simulink library "gavrt_library"  (Simulink 7.1)
undefined symbols (not defined in the file or in its folder): Convert, Counter, Mux, xbsIndex_r3
libraries: xbsIndex_r4 x210, xps_library x15, casper_library x12, gavrt_library x8, xbsReplacements_r4 x7
(part 2 of 3)

== system gavrt_library/commutator ==
  reset : Inport  OutDataType=sfix(16)  OutScaling=2^0
  enable : Inport  Port=2  OutDataType=sfix(16)  OutScaling=2^0
  din : Inport  Port=3  OutDataType=sfix(16)  OutScaling=2^0
  Mux : S-Function  AncestorBlock=xbsIndex_r3/Mux  FunctionName=xlmux  Parameters=sfcn_mwsv__  EnableBusSupport=off  mask(Xilinx Multiplexer Block){inputs=8, precision=Full, arith_type=Signed  (2's comp), n_bits=8, bin_pt=2, quantization=Truncate, overflow=Wrap, latency=2, explicit_period=off, period=1, en=off, dbl_ovrd=off, show_param=off, mux_type=off, use_rpm=off, gen_core=off, xl_area=[0, 0, 0, 0, 0, 0, 0], xl_use_area=off}
      mask prompts: inputs "Number of Inputs"; arith_type "Arithmetic Type"; n_bits "Number of Bits"; bin_pt "Binary Point"; explicit_period "Use Explicit Sample Period"; period "Sample Period  (use -1 to inherit first known input period)"; en "Provide Enable Port"; dbl_ovrd "Override with Doubles"; show_param "---------------------- Show Implementation Parameters -----------------------------------------------------------------------------------"; mux_type "Use Tristate Buffers"; use_rpm "Use Placement Information for Core"; gen_core "Generate Core"; xl_area "FPGA Area [Slices, FFs, BRAMs, LUTs, IOBs, Emb. Mults, TBUFs]"; xl_use_area "Use Area Above For Estimation"
      mask help:
      | Bus Multiplexer.  Binary points are aligned automatically.
      |
      | Hardware notes: A multiplexer using tristate buffers requires fewer lookup tables but is slower.
      mask init:
      | [designRoot, family, part, speed, package, simulinkPeriod, sysclkPeriod, dbl_ovrd, trimVbit] = xlSysgenSettings(gcb,1,1);
      | num_inputs = inputs+1;
      | [bg,fg] = xlcmap('XBlock',dbl_ovrd);
      | zstr='';
      | zpstr='';
      | if latency > 0
      |   zstr = 'z';
      |   zpstr = sprintf('-%d', latency);
      | end
      | 
      | dprt = [2:inputs+2 2+zeros(1,32-inputs)];
      | dstr0 = 'd0';
      | dstr1 = 'd1';
      | dstr2='';dstr3='';dstr4='';dstr5='';dstr6='';dstr7='';dstr8='';dstr9='';dstr10='';
      | dstr11='';dstr12='';dstr12='';dstr13='';dstr14='';dstr15='';dstr16='';dstr17='';dstr18='';dstr19='';dstr20='';dstr21='';dstr22='';dstr23='';dstr24='';dstr25='';dstr26='';dstr27='';dstr28='';dstr29='';dstr30='';dstr31='';
      | 
      | if (inputs>=2) dstr2 = 'd2'; end
      | if (inputs>=3) dstr3 = 'd3'; end
      | if (inputs>=4) dstr4 = 'd4'; end
      | if (inputs>=5) dstr5 = 'd5'; end
      | if (inputs>=6) dstr6 = 'd6'; end
      | if (inputs>=7) dstr7 = 'd7'; end
      | if (inputs>=8) dstr8 = 'd8'; end
      | if (inputs>=9) dstr9 = 'd9'; end
      | if (inputs>=10) dstr10 = 'd10'; end
      | if (inputs>=11) dstr11 = 'd11'; end
      | if (inputs>=12) dstr12 = 'd12'; end
      | if (inputs>=13) dstr13 = 'd13'; end
      | if (inputs>=14) dstr14 = 'd14'; end
      | if (inputs>=15) dstr15 = 'd15'; end
      | if (inputs>=16) dstr16 = 'd16'; end
      | if (inputs>=17) dstr17 = 'd17'; end
      | if (inputs>=18) dstr18 = 'd18'; end
      | if (inputs>=19) dstr19 = 'd19'; end
      | if (inputs>=20) dstr20 = 'd20'; end
      | if (inputs>=21) dstr21 = 'd21'; end
      | if (inputs>=22) dstr22 = 'd22'; end
      | if (inputs>=23) dstr23 = 'd23'; end
      | if (inputs>=24) dstr24 = 'd24'; end
      | if (inputs>=25) dstr25 = 'd25'; end
      | if (inputs>=26) dstr26 = 'd26'; end
      | if (inputs>=27) dstr27 = 'd27'; end
      | if (inputs>=28) dstr28 = 'd28'; end
      | if (inputs>=29) dstr29 = 'd29'; end
      | if (inputs>=30) dstr30 = 'd30'; end
      | if (inputs>=31) dstr31 = 'd31'; end
      | 
      | iPos = get_param(gcb,'Position');
      | iWidth=iPos(3)-iPos(1); iHeight=iPos(4)-iPos(2);
      | iCx=iWidth/2;
      | iCy=iHeight/2;
      | [logoX, logoY] = xlogo(iPos);
      | 
      | rst = 0;
      | [enPortNum, enPortStr, rstPortNum, rstPortStr, portDir] = xlport_en_rst(en, rst, num_inputs+2);
      | % one time added for param list
      | hasEN = en;
      | hasRST = rst;
      | dblOvrd = dbl_ovrd;
      | numInputs = num_inputs;
      | muxType = mux_type;
      | useCore = 1;
      | precision0 = precision;
      | z0 = [n_bits  bin_pt arith_type quantization overflow];
      | explicitClk = explicit_period;
      | gen_core = 1;
      | 
      | % just pass everything to s-function
      | sfcn_mwsv__ = get_param(gcb, 'MaskWSVariables');
      mask Help: eval('xlWeb(xlhtmldoclink(''Mux''))');
      mask StyleString: popup(2|3|4|5|6|7|8|9|10|11|12|13|14|15|16|17|18|19|20|21|22|23|24|25|26|27|28|29|30|31|32),popup(Full|User Defined),popup(Unsigned|Signed  (2's comp)),edit,edit,popup(Truncate|Round  (unbiased: +/- Inf)),popup(Wrap|Saturate|Flag as Error),edit,checkbox,edit,checkbox,checkbox,checkbox,checkbox,checkbox,checkbox,edit,checkbox
      mask CallbackString: |xlMagicCallback|||||||xlMagicCallback||||xlShowIPCallback|||||
      mask Display:
      | patch([0 iWidth iWidth 0],[0 1/7*iHeight 6/7*iHeight iHeight] , bg);
      | patch(logoX,logoY, fg);
      | plot([0 iWidth iWidth 0 0],[0 1/7*iHeight 6/7*iHeight iHeight 0] );
      | text(iCx-5,iCy-5,zstr);
      | text(iCx,iCy,zpstr);
      | port_label('input',1,'sel');
      | port_label('input',dprt(1),dstr0);
      | port_label('input',dprt(2),dstr1);
      | port_label('input',dprt(2),dstr1);
      | port_label('input',dprt(3),dstr2);
      | port_label('input',dprt(4),dstr3);
      | port_label('input',dprt(5),dstr4);
      | port_label('input',dprt(6),dstr5);
      | port_label('input',dprt(7),dstr6);
      | port_label('input',dprt(8),dstr7);
      | port_label('input',dprt(9),dstr8);
      | port_label('input',dprt(10),dstr9);
      | port_label('input',dprt(11),dstr10);
      | port_label('input',dprt(12),dstr11);
      | port_label('input',dprt(13),dstr12);
      | port_label('input',dprt(14),dstr13);
      | port_label('input',dprt(15),dstr14);
      | port_label('input',dprt(16),dstr15);
      | port_label('input',dprt(17),dstr16);
      | port_label('input',dprt(18),dstr17);
      | port_label('input',dprt(19),dstr18);
      | port_label('input',dprt(20),dstr19);
      | port_label('input',dprt(21),dstr20);
      | port_label('input',dprt(22),dstr21);
      | port_label('input',dprt(23),dstr22);
      | port_label('input',dprt(24),dstr23);
      | port_label('input',dprt(25),dstr24);
      | port_label('input',dprt(26),dstr25);
      | port_label('input',dprt(27),dstr26);
      | port_label('input',dprt(28),dstr27);
      | port_label('input',dprt(29),dstr28);
      | port_label('input',dprt(30),dstr29);
      | port_label('input',dprt(31),dstr30);
      | port_label('input',dprt(32),dstr31);
      | port_label(portDir,enPortNum,enPortStr);
  index_cnt : S-Function  AncestorBlock=xbsIndex_r3/Counter  FunctionName=xlcounter  Parameters=sfcn_mwsv__  EnableBusSupport=off  mask(Xilinx Counter Block){cnt_type=Free Running, n_bits=3, bin_pt=0, arith_type=Unsigned, start_count=0, cnt_to=Inf, cnt_by_val=1, operation=Up, explicit_period=off, period=1, load_pin=off, rst=on, en=on, dbl_ovrd=off, show_param=off, use_rpm=on, gen_core=off, xl_area=[0, 0, 0, 0, 0, 0, 0], xl_use_area=off}
      mask prompts: cnt_type "Counter Type"; n_bits "Number of Bits"; bin_pt "Binary Point Position"; arith_type "Arithmetic Type"; start_count "Initial Value"; cnt_to "Count To Value"; cnt_by_val "Step"; operation "Count Direction"; explicit_period "Use Explicit Sample Period"; period "Sample Period"; load_pin "Provide Load Port"; rst "Provide Reset Port"; en "Provide Enable Port"; dbl_ovrd "Override with Doubles"; show_param "---------------------- Show Implementation Parameters -----------------------------------------------------------------------------------"; use_rpm "Use Placement Information for Core"; gen_core "Generate Core"; xl_area "FPGA Area [Slices, FFs, BRAMs, LUTs, IOBs, Emb. Mults, TBUFs]"; xl_use_area "Use Area Above For Estimation"
      mask help:
      | Configurable up, down and up/down counter.
      |
      | Hardware notes: Free running counters are the least expensive in hardware.  A count limited counter is implemented by combining a counter with a comparator.
      mask init:
      | if ((rst==1) | (en==1) | (operation == 3) | ( (cnt_type == 2)&(load_pin == 1)))
      |   explicitClk = explicit_period;
      | else
      |   explicitClk =1;
      | end
      | numinputs = 0;
      | upDir = 'output';
      | upPNum = 1;
      | upStr = '';
      | loadDir = 'output';
      | loadPNum = 1;
      | loadStr = '';
      | dinDir = 'output';
      | dinPNum = 1;
      | dinStr = '';
      | if (operation == 3)
      |    numinputs = numinputs + 1;
      |    upDir = 'input';
      |   upPNum = numinputs;
      |    upStr = 'up';
      | end
      | 
      | if (cnt_type == 2)
      |   if (load_pin)
      |     loadDir = 'input';
      |     loadStr = 'load';
      |     numinputs = numinputs + 1;
      |     loadPNum = numinputs;
      |     dinDir = 'input';
      |     dinStr = 'din';
      |     numinputs = numinputs + 1;
      |     dinPNum = numinputs;
      |  end
      | end
      | numinputs = numinputs + 1;
      | [designRoot, family, part, speed, package, simulinkPeriod, sysclkPeriod, dbl_ovrd, trimVbit] = xlSysgenSettings(gcb,1,1);
      | [enPortNum, enPortStr, rstPortNum, rstPortStr, portDir] = xlport_en_rst(en, rst, numinputs);
      | [bg,fg]=xlcmap('XBlock',dbl_ovrd);
      | iPos = get_param(gcb,'Position');
      | iWidth=iPos(3)-iPos(1); iHeight=iPos(4)-iPos(2);
      | iCx=iWidth/2;
      | iCy=iHeight/2;
      | [logoX, logoY] = xlogo(iPos);
      | 
      | 
      | % one time added for param list
      | dblOvrd = dbl_ovrd;
      | precision0 = 2;
      | z0 = [n_bits bin_pt arith_type  1 1];
      | hasEN = en;
      | hasRST = rst;
      | hasLoad = load_pin;
      | latency = 1;
      | useCore = 1;
      | gen_core = 1;
      | 
      | % just pass everything to s-function
      | sfcn_mwsv__ = get_param(gcb, 'MaskWSVariables');
      mask Help: eval('xlWeb(xlhtmldoclink(''Counter''))');
      mask StyleString: popup(Count Limited|Free Running),edit,edit,popup(Unsigned|Signed  (2's comp)),edit,edit,edit,popup(Up|Down|Up/Down),checkbox,edit,checkbox,checkbox,checkbox,checkbox,checkbox,checkbox,checkbox,edit,checkbox
      mask CallbackString: xlcounterCallback|||||||xlcounterCallback|xlcounterCallback||xlcounterCallback|xlcounterCallback|xlcounterCallback||xlShowIPCallback||||
      mask Display:
      | patch([0 iWidth iWidth 0],[0 0 iHeight iHeight] , bg);
      | patch(logoX,logoY , fg);
      | port_label('output',1,'out');
      | port_label(upDir,upPNum,upStr);
      | port_label(dinDir,dinPNum,dinStr);
      | port_label(loadDir,loadPNum,loadStr);
      | port_label(portDir,rstPortNum,rstPortStr);
      | port_label(portDir,enPortNum,enPortStr);
      | plot([0 0 iWidth iWidth 0], [0 iHeight iHeight 0 0]);
  uncram : gavrt_library/uncram  SystemSampleTime=-1  num_slice=8  slice_width=32  bin_pt=0  arith_type=0
      settings: AttributesFormatString=UFix_32_0
  index : Outport  Orientation=up  OutDataType=sfix(16)  OutScaling=2^0
  dout : Outport  Port=2  OutDataType=sfix(16)  OutScaling=2^0
  wires:
  reset/1 -> index_cnt/1
  enable/1 -> index_cnt/2
  din/1 -> uncram/1
  index_cnt/1 -> index/1, Mux/1
  Mux/1 -> dout/1
  uncram/1 -> Mux/2
  uncram/2 -> Mux/3
  uncram/3 -> Mux/4
  uncram/4 -> Mux/5
  uncram/5 -> Mux/6
  uncram/6 -> Mux/7
  uncram/7 -> Mux/8
  uncram/8 -> Mux/9

== system gavrt_library/cram ==
  In1 : Inport  OutDataType=sfix(16)  OutScaling=2^0
  In2 : Inport  Port=2  OutDataType=sfix(16)  OutScaling=2^0
  In3 : Inport  Port=3  OutDataType=sfix(16)  OutScaling=2^0
  In4 : Inport  Port=4
  Concat : xbsIndex_r4/Concat  num_inputs=4  dbl_ovrd=off  block_type=concat
      settings: block_version=10.1.2
  Reinterp{1..4} (4 alike) : xbsIndex_r4/Reinterpret  force_arith_type=on  arith_type=Unsigned  force_bin_pt=on  bin_pt=0  block_type=reinterpret
      settings: infoedit="Changes signal type without altering the binary representation.   You can changed the signal between signed and unsigned, and relocate the binary point.<P><P>Hardware notes: In hardware this block costs nothing.<P><P>Example:  Suppose the input is 6 bits wide, signed, with 2 fractional bits, and the output is forced to unsigned with 0 fractional bits.  Then an input of -2.0 (1110.00 in binary 2's complement) becomes an output of 56 (111000 in binary)."  block_version=10.1.2
  Out : Outport
  wires:
  Reinterp4/1 -> Concat/4
  In4/1 -> Reinterp4/1
  Reinterp3/1 -> Concat/3
  In3/1 -> Reinterp3/1
  Reinterp2/1 -> Concat/2
  In2/1 -> Reinterp2/1
  Reinterp1/1 -> Concat/1
  In1/1 -> Reinterp1/1
  Concat/1 -> Out/1

== system gavrt_library/fpga_cplx_to_sim_cplx ==
  in : Inport  OutDataType=sfix(16)  OutScaling=2^0
  Gateway Out10 : xbsIndex_r4/Gateway Out  hdl_port=on  timing_constraint=None  locs_specified=off  LOCs={}  block_type=gatewayout
      settings: infoedit="Gateway out block.  Converts Xilinx fixed point inputs into ouputs of type Simulink integer, double, or fixed point.<P><P>Hardware notes:  In hardware these blocks become top level output ports or are discarded, depending on how they are configured."  xl_area=[0, 0, 0, 0, 0, 0, 0]  block_version=10.1.2
  Gateway Out6 : xbsIndex_r4/Gateway Out  hdl_port=on  timing_constraint=None  locs_specified=off  LOCs={}  block_type=gatewayout
      settings: infoedit="Gateway out block.  Converts Xilinx fixed point inputs into ouputs of type Simulink integer, double, or fixed point.<P><P>Hardware notes:  In hardware these blocks become top level output ports or are discarded, depending on how they are configured."  xl_area=[0, 0, 0, 0, 0, 0, 0]  block_version=10.1.2
  Real-Imag to Complex : RealImagToComplex
  c_to_ri : casper_library/Misc/c_to_ri  SystemSampleTime=-1  n_bits=width  bin_pt=width-1
      settings: AttributesFormatString=18_17 r/i
  cplx : Outport  OutDataType=sfix(16)  OutScaling=2^0
  re : Outport  Port=2  OutDataType=sfix(16)  OutScaling=2^0
  im : Outport  Port=3  OutDataType=sfix(16)  OutScaling=2^0
  wires:
  c_to_ri/1 -> Gateway Out6/1
  c_to_ri/2 -> Gateway Out10/1
  Gateway Out6/1 -> Real-Imag to Complex/1, re/1
  Gateway Out10/1 -> Real-Imag to Complex/2, im/1
  Real-Imag to Complex/1 -> cplx/1
  in/1 -> c_to_ri/1

== system gavrt_library/nCasts ==
  In1 : Inport  OutDataType=sfix(16)  OutScaling=2^0
  In2 : Inport  Port=2  OutDataType=sfix(16)  OutScaling=2^0
  Cast1 : xbsIndex_r4/Convert  arith_type=Unsigned  n_bits=8  bin_pt=3  quantization=Truncate  overflow=Wrap  latency=0  dbl_ovrd=off  pipeline=off  block_type=convert
      settings: xl_area=[0, 0, 0, 0, 0, 0, 0]  block_version=10.1.2
  Cast2 : xbsIndex_r4/Convert  arith_type=Unsigned  n_bits=8  bin_pt=3  quantization=Truncate  overflow=Wrap  latency=0  dbl_ovrd=off  pipeline=off  block_type=convert
      settings: xl_area=[0, 0, 0, 0, 0, 0, 0]  block_version=10.1.2
  Out1 : Outport  OutDataType=sfix(16)  OutScaling=2^0
  Out2 : Outport  Port=2  OutDataType=sfix(16)  OutScaling=2^0
  wires:
  Cast2/1 -> Out2/1
  In2/1 -> Cast2/1
  Cast1/1 -> Out1/1
  In1/1 -> Cast1/1

== system gavrt_library/npower ==
  sync_in : Inport  OutDataType=sfix(16)  OutScaling=2^0
  din1 : Inport  Port=2  OutDataType=sfix(16)  OutScaling=2^0
  din2 : Inport  Port=3  OutDataType=sfix(16)  OutScaling=2^0
  power1 : gavrt_library/power  SystemSampleTime=-1  BitWidth=18  add_latency=2  mult_latency=3
  power2 : gavrt_library/power  SystemSampleTime=-1  BitWidth=18  add_latency=2  mult_latency=3
  sync_delay : xbsIndex_r4/Delay  en=off  latency=5  dbl_ovrd=off  reg_retiming=off  block_type=delay
      settings: xl_area=[0, 0, 0, 0, 0, 0, 0]  block_version=10.1.2
  sync_out : Outport  OutDataType=sfix(16)  OutScaling=2^0
  dout1 : Outport  Port=2  OutDataType=sfix(16)  OutScaling=2^0
  dout2 : Outport  Port=3  OutDataType=sfix(16)  OutScaling=2^0
  wires:
  sync_in/1 -> sync_delay/1
  sync_delay/1 -> sync_out/1
  din1/1 -> power1/1
  power1/1 -> dout1/1
  din2/1 -> power2/1
  power2/1 -> dout2/1

== system gavrt_library/pow ==
  cplx : Inport  OutDataType=sfix(16)  OutScaling=2^0
  c_to_ri : casper_library/Misc/c_to_ri  SystemSampleTime=-1  n_bits=bit_width  bin_pt=bit_width - 1
      settings: AttributesFormatString=_ r/i
  imag_square : xbsIndex_r4/Mult  precision=Full  arith_type="Signed  (2's comp)"  n_bits=8  bin_pt=2  quantization=Truncate  overflow=Wrap  en=off  latency=mult_latency  dbl_ovrd=off  use_behavioral_HDL=off  use_embedded=on  opt=Speed  optimum_pipeline=off  pipeline=on  use_rpm=on  placement_style=Rectangular shape  block_type=mult
      settings: infoedit=Hardware notes: To use the internal pipeline stage of the dedicated multiplier you must select 'Pipeline for maximum performance'.  xl_area=[0, 0, 0, 0, 0, 0, 0]  block_version=10.1.2
  power_adder : xbsIndex_r4/AddSub  mode=Addition  use_carryin=off  use_carryout=off  en=off  latency=add_latency  precision=User Defined  arith_type=Unsigned  n_bits=bit_width * 2  bin_pt=bit_width * 2 - 1  quantization=Truncate  overflow=Wrap  dbl_ovrd=off  use_behavioral_HDL=on  pipelined=off  use_rpm=on  block_type=addsub
      settings: xl_area=[0, 0, 0, 0, 0, 0, 0]  block_version=10.1.2
  real_square : xbsIndex_r4/Mult  precision=Full  arith_type="Signed  (2's comp)"  n_bits=8  bin_pt=2  quantization=Truncate  overflow=Wrap  en=off  latency=mult_latency  dbl_ovrd=off  use_behavioral_HDL=off  use_embedded=on  opt=Speed  optimum_pipeline=off  pipeline=on  use_rpm=on  placement_style=Rectangular shape  block_type=mult
      settings: infoedit=Hardware notes: To use the internal pipeline stage of the dedicated multiplier you must select 'Pipeline for maximum performance'.  xl_area=[0, 0, 0, 0, 0, 0, 0]  block_version=10.1.2
  magsq : Outport  OutDataType=sfix(16)  OutScaling=2^0
  wires:
  imag_square/1 -> power_adder/2
  real_square/1 -> power_adder/1
  c_to_ri/1 -> real_square/1, real_square/2
  c_to_ri/2 -> imag_square/2, imag_square/1
  cplx/1 -> c_to_ri/1
  power_adder/1 -> magsq/1

== system gavrt_library/power ==
  c : Inport  OutDataType=sfix(16)  OutScaling=2^0
  c_to_ri : casper_library/Misc/c_to_ri  SystemSampleTime=-1  n_bits=BitWidth  bin_pt=BitWidth-1
      settings: AttributesFormatString=_ r/i
  imag_square : xbsIndex_r4/Mult  precision=Full  arith_type="Signed  (2's comp)"  n_bits=8  bin_pt=2  quantization=Truncate  overflow=Wrap  en=off  latency=mult_latency  dbl_ovrd=off  use_behavioral_HDL=off  use_embedded=on  opt=Speed  optimum_pipeline=off  pipeline=on  use_rpm=on  placement_style=Rectangular shape  block_type=mult
      settings: infoedit=Hardware notes: To use the internal pipeline stage of the dedicated multiplier you must select 'Pipeline for maximum performance'.  xl_area=[0, 0, 0, 0, 0, 0, 0]  block_version=10.1.2
  power_adder : xbsIndex_r4/AddSub  mode=Addition  use_carryin=off  use_carryout=off  en=off  latency=add_latency  precision=User Defined  arith_type=Unsigned  n_bits=2*BitWidth  bin_pt=2*BitWidth-1  quantization=Truncate  overflow=Wrap  dbl_ovrd=off  use_behavioral_HDL=on  pipelined=off  use_rpm=on  block_type=addsub
      settings: xl_area=[0, 0, 0, 0, 0, 0, 0]  block_version=10.1.2
  real_square : xbsIndex_r4/Mult  precision=Full  arith_type="Signed  (2's comp)"  n_bits=8  bin_pt=2  quantization=Truncate  overflow=Wrap  en=off  latency=mult_latency  dbl_ovrd=off  use_behavioral_HDL=off  use_embedded=on  opt=Speed  optimum_pipeline=off  pipeline=on  use_rpm=on  placement_style=Rectangular shape  block_type=mult
      settings: infoedit=Hardware notes: To use the internal pipeline stage of the dedicated multiplier you must select 'Pipeline for maximum performance'.  xl_area=[0, 0, 0, 0, 0, 0, 0]  block_version=10.1.2
  power : Outport  OutDataType=sfix(16)  OutScaling=2^0
  wires:
  c_to_ri/2 -> imag_square/1, imag_square/2
  c_to_ri/1 -> real_square/2, real_square/1
  c/1 -> c_to_ri/1
  real_square/1 -> power_adder/1
  imag_square/1 -> power_adder/2
  power_adder/1 -> power/1

== system gavrt_library/sim_cplx_to_fpga_cplx ==
  sim : Inport  OutDataType=sfix(16)  OutScaling=2^0
  Complex to Real-Imag : ComplexToRealImag
  Gateway In1 : xbsIndex_r4/Gateway In  arith_type="Signed  (2's comp)"  n_bits=width  bin_pt=width-1  quantization=Truncate  overflow=Wrap  period=1  dbl_ovrd=off  timing_constraint=None  locs_specified=off  LOCs={}  block_type=gatewayin
      settings: infoedit="Gateway in block.  Converts inputs of type Simulink integer, double and fixed point to  Xilinx fixed point type.<P><P>Hardware notes:  In hardware these blocks become top level input ports."  xl_area=[0, 0, 0, 0, 0, 0, 0]  block_version=10.1.2
  Gateway In2 : xbsIndex_r4/Gateway In  arith_type="Signed  (2's comp)"  n_bits=width  bin_pt=width-1  quantization=Truncate  overflow=Wrap  period=1  dbl_ovrd=off  timing_constraint=None  locs_specified=off  LOCs={}  block_type=gatewayin
      settings: infoedit="Gateway in block.  Converts inputs of type Simulink integer, double and fixed point to  Xilinx fixed point type.<P><P>Hardware notes:  In hardware these blocks become top level input ports."  xl_area=[0, 0, 0, 0, 0, 0, 0]  block_version=10.1.2
  ri_to_c : casper_library/Misc/ri_to_c  SystemSampleTime=-1
  fpga : Outport  OutDataType=sfix(16)  OutScaling=2^0
  wires:
  Complex to Real-Imag/1 -> Gateway In1/1
  Complex to Real-Imag/2 -> Gateway In2/1
  Gateway In1/1 -> ri_to_c/1
  Gateway In2/1 -> ri_to_c/2
  ri_to_c/1 -> fpga/1
  sim/1 -> Complex to Real-Imag/1

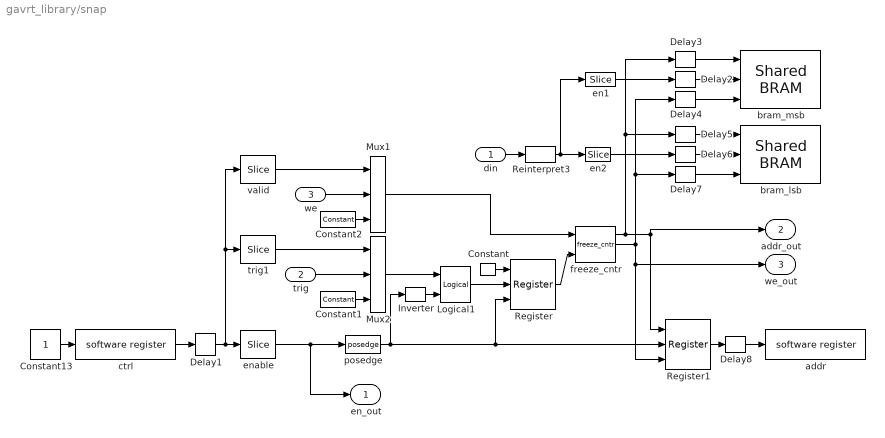
== system gavrt_library/snap ==
  din : Inport  OutDataType=sfix(16)  OutScaling=2^0
  trig : Inport  Port=2  OutDataType=sfix(16)  OutScaling=2^0
  we : Inport  Port=3  OutDataType=sfix(16)  OutScaling=2^0
  Constant : xbsIndex_r4/Constant  arith_type=Boolean  const=1  n_bits=1  bin_pt=0  explicit_period=on  period=1  equ=P=C  opselect=C  inp2=PCIN>>17  opr=+  inp1=P  carry=CIN  dbl_ovrd=off  block_type=constant
      settings: block_version=10.1.2
  Constant1 : xbsIndex_r4/Constant  arith_type=Boolean  const=1  n_bits=1  bin_pt=0  explicit_period=on  period=1  equ=P=C  opselect=C  inp2=PCIN>>17  opr=+  inp1=P  carry=CIN  dbl_ovrd=off  block_type=constant
      settings: block_version=10.1.2
  Constant13 : Constant  OutDataType=sfix(16)  OutScaling=2^0
  Constant2 : xbsIndex_r4/Constant  arith_type=Boolean  const=1  n_bits=1  bin_pt=0  explicit_period=on  period=1  equ=P=C  opselect=C  inp2=PCIN>>17  opr=+  inp1=P  carry=CIN  dbl_ovrd=off  block_type=constant
      settings: block_version=10.1.2
  Delay{1..8} (8 alike) : xbsIndex_r4/Delay  en=off  latency=latency  dbl_ovrd=off  reg_retiming=on  block_type=delay
      settings: xl_area=[0, 0, 0, 0, 0, 0, 0]  block_version=10.1.2
  Inverter : xbsIndex_r4/Inverter  en=off  latency=0  dbl_ovrd=off  block_type=inv
      settings: xl_area=[0, 0, 0, 0, 0, 0, 0]  block_version=10.1.2
  Logical1 : xbsIndex_r4/Logical  logical_function=AND  inputs=2  en=off  latency=0  precision=Full  arith_type=Unsigned  n_bits=8  bin_pt=2  align_bp=on  dbl_ovrd=off  block_type=logical
      settings: xl_area=[0, 0, 0, 0, 0, 0, 0]  block_version=10.1.2
  Mux1 : xbsIndex_r4/Mux  inputs=2  en=off  latency=0  precision=Full  arith_type="Signed  (2's comp)"  n_bits=8  bin_pt=2  quantization=Truncate  overflow=Wrap  dbl_ovrd=off  block_type=mux
      settings: xl_area=[0, 0, 0, 0, 0, 0, 0]  block_version=10.1.2
  Mux2 : xbsIndex_r4/Mux  inputs=2  en=off  latency=0  precision=Full  arith_type="Signed  (2's comp)"  n_bits=8  bin_pt=2  quantization=Truncate  overflow=Wrap  dbl_ovrd=off  block_type=mux
      settings: xl_area=[0, 0, 0, 0, 0, 0, 0]  block_version=10.1.2
  Register : xbsIndex_r4/Register  init=0  rst=on  en=on  dbl_ovrd=off  block_type=register
      settings: xl_area=[0, 0, 0, 0, 0, 0, 0]  block_version=10.1.2
  Register1 : xbsIndex_r4/Register  init=0  rst=on  en=on  dbl_ovrd=off  block_type=register
      settings: xl_area=[0, 0, 0, 0, 0, 0, 0]  block_version=10.1.2
  Reinterpret3 : xbsIndex_r4/Reinterpret  force_arith_type=on  arith_type=Unsigned  force_bin_pt=on  bin_pt=0  block_type=reinterpret
      settings: infoedit="Changes signal type without altering the binary representation.   You can changed the signal between signed and unsigned, and relocate the binary point.<P><P>Hardware notes: In hardware this block costs nothing.<P><P>Example:  Suppose the input is 6 bits wide, signed, with 2 fractional bits, and the output is forced to unsigned with 0 fractional bits.  Then an input of -2.0 (1110.00 in binary 2's complement) becomes an output of 56 (111000 in binary)."  block_version=10.1.2
  addr : xps_library/software register  Tag=xps:sw_reg  SystemSampleTime=-1  io_dir=To Processor  arith_type=Unsigned  bitwidth=32  bin_pt=0  sample_period=1  gw_name=gavrt_library_snap_addr_user_data_in
  bram_lsb : xps_library/Shared BRAM  Tag=xps:bram  SystemSampleTime=-1  arith_type=Unsigned  addr_width=nsamples  data_width=32  data_bin_pt=0  init_vals=0  sample_rate=1
  bram_msb : xps_library/Shared BRAM  Tag=xps:bram  SystemSampleTime=-1  arith_type=Unsigned  addr_width=nsamples  data_width=32  data_bin_pt=0  init_vals=0  sample_rate=1
  ctrl : xps_library/software register  Tag=xps:sw_reg  SystemSampleTime=-1  io_dir=From Processor  arith_type=Unsigned  bitwidth=32  bin_pt=0  sample_period=1  gw_name=gavrt_library_snap_ctrl_user_data_out
  en1 : xbsIndex_r4/Slice  nbits=32  boolean_output=off  mode=Lower Bit Location + Width  bit1=0  base1=LSB of Input  bit0=32  base0=LSB of Input  dbl_ovrd=off  block_type=slice
      settings: infoedit="Extracts a given range of bits from each input sample and presents it at the output.  The output type is ordinarily unsigned with binary point at zero, but can be Boolean when the slice is one bit wide.<P><P>Hardware notes: In hardware this block costs nothing."  block_version=10.1.2
  en2 : xbsIndex_r4/Slice  nbits=32  boolean_output=off  mode=Lower Bit Location + Width  bit1=0  base1=LSB of Input  bit0=0  base0=LSB of Input  dbl_ovrd=off  block_type=slice
      settings: infoedit="Extracts a given range of bits from each input sample and presents it at the output.  The output type is ordinarily unsigned with binary point at zero, but can be Boolean when the slice is one bit wide.<P><P>Hardware notes: In hardware this block costs nothing."  block_version=10.1.2
  enable : xbsIndex_r4/Slice  nbits=1  boolean_output=on  mode=Lower Bit Location + Width  bit1=0  base1=LSB of Input  bit0=0  base0=LSB of Input  dbl_ovrd=off  block_type=slice
      settings: infoedit="Extracts a given range of bits from each input sample and presents it at the output.  The output type is ordinarily unsigned with binary point at zero, but can be Boolean when the slice is one bit wide.<P><P>Hardware notes: In hardware this block costs nothing."  block_version=10.1.2
  freeze_cntr : casper_library/Misc/freeze_cntr  SystemSampleTime=-1  CounterBits=nsamples
  posedge : casper_library/Misc/posedge  Tag=Rising Edge Detector  SystemSampleTime=-1
  trig1 : xbsIndex_r4/Slice  nbits=1  boolean_output=on  mode=Lower Bit Location + Width  bit1=0  base1=LSB of Input  bit0=1  base0=LSB of Input  dbl_ovrd=off  block_type=slice
      settings: infoedit="Extracts a given range of bits from each input sample and presents it at the output.  The output type is ordinarily unsigned with binary point at zero, but can be Boolean when the slice is one bit wide.<P><P>Hardware notes: In hardware this block costs nothing."  block_version=10.1.2
  valid : xbsIndex_r4/Slice  nbits=1  boolean_output=on  mode=Lower Bit Location + Width  bit1=0  base1=LSB of Input  bit0=2  base0=LSB of Input  dbl_ovrd=off  block_type=slice
      settings: infoedit="Extracts a given range of bits from each input sample and presents it at the output.  The output type is ordinarily unsigned with binary point at zero, but can be Boolean when the slice is one bit wide.<P><P>Hardware notes: In hardware this block costs nothing."  block_version=10.1.2
  en_out : Outport  OutDataType=sfix(16)  OutScaling=2^0
  addr_out : Outport  Port=2  OutDataType=sfix(16)  OutScaling=2^0
  we_out : Outport  Port=3  OutDataType=sfix(16)  OutScaling=2^0
  wires:
  Delay7/1 -> bram_lsb/3
  Delay6/1 -> bram_lsb/2
  Delay5/1 -> bram_lsb/1
  Delay4/1 -> bram_msb/3
  Delay2/1 -> bram_msb/2
  Delay3/1 -> bram_msb/1
  Delay8/1 -> addr/1
  Delay1/1 -> enable/1, valid/1, trig1/1
  en2/1 -> Delay6/1
  en1/1 -> Delay2/1
  din/1 -> Reinterpret3/1
  Reinterpret3/1 -> en2/1, en1/1
  trig/1 -> Mux2/2
  enable/1 -> en_out/1, posedge/1
  freeze_cntr/2 -> we_out/1, Register1/3, Delay7/1, Delay4/1
  Constant13/1 -> ctrl/1
  ctrl/1 -> Delay1/1
  posedge/1 -> Register/3, Register1/2, Inverter/1
  Constant/1 -> Register/1
  Constant1/1 -> Mux2/3
  Mux1/1 -> freeze_cntr/1
  we/1 -> Mux1/2
  Constant2/1 -> Mux1/3
  Register1/1 -> Delay8/1
  trig1/1 -> Mux2/1
  valid/1 -> Mux1/1
  Logical1/1 -> Register/2
  Inverter/1 -> Logical1/2
  Mux2/1 -> Logical1/1
  Register/1 -> freeze_cntr/2
  freeze_cntr/1 -> addr_out/1, Register1/1, Delay5/1, Delay3/1

== system gavrt_library/supercat ==
  i1 : Inport  OutDataType=sfix(16)  OutScaling=2^0
  i2 : Inport  Port=2  OutDataType=sfix(16)  OutScaling=2^0
  i3 : Inport  Port=3  OutDataType=sfix(16)  OutScaling=2^0
  i4 : Inport  Port=4  OutDataType=sfix(16)  OutScaling=2^0
  i5 : Inport  Port=5  OutDataType=sfix(16)  OutScaling=2^0
  i6 : Inport  Port=6  OutDataType=sfix(16)  OutScaling=2^0
  i7 : Inport  Port=7  OutDataType=sfix(16)  OutScaling=2^0
  i8 : Inport  Port=8  OutDataType=sfix(16)  OutScaling=2^0
  Concat_1 : xbsIndex_r4/Concat  num_inputs=8  dbl_ovrd=off  block_type=concat
      settings: block_version=10.1.2
  Out : Outport  OutDataType=sfix(16)  OutScaling=2^0
  wires:
  i1/1 -> Concat_1/1
  i2/1 -> Concat_1/2
  i3/1 -> Concat_1/3
  i4/1 -> Concat_1/4
  i5/1 -> Concat_1/5
  i6/1 -> Concat_1/6
  i7/1 -> Concat_1/7
  i8/1 -> Concat_1/8
  Concat_1/1 -> Out/1

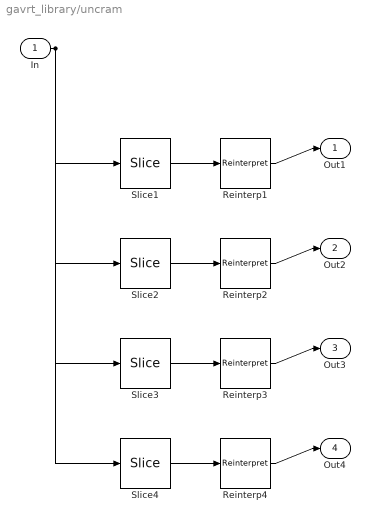
== system gavrt_library/uncram ==
  In : Inport  OutDataType=sfix(16)  OutScaling=2^0
  Reinterp{1..4} (4 alike) : xbsIndex_r4/Reinterpret  force_arith_type=on  arith_type="Signed  (2's comp)"  force_bin_pt=on  bin_pt=17  block_type=reinterpret
      settings: infoedit="Changes signal type without altering the binary representation.   You can changed the signal between signed and unsigned, and relocate the binary point.<P><P>Hardware notes: In hardware this block costs nothing.<P><P>Example:  Suppose the input is 6 bits wide, signed, with 2 fractional bits, and the output is forced to unsigned with 0 fractional bits.  Then an input of -2.0 (1110.00 in binary 2's complement) becomes an output of 56 (111000 in binary)."  block_version=10.1.2
  Slice1 : xbsIndex_r4/Slice  nbits=18  boolean_output=off  mode=Upper Bit Location + Width  bit1=0  base1=MSB of Input  bit0=0  base0=LSB of Input  dbl_ovrd=off  block_type=slice
      settings: infoedit="Extracts a given range of bits from each input sample and presents it at the output.  The output type is ordinarily unsigned with binary point at zero, but can be Boolean when the slice is one bit wide.<P><P>Hardware notes: In hardware this block costs nothing."  block_version=10.1.2
  Slice2 : xbsIndex_r4/Slice  nbits=18  boolean_output=off  mode=Upper Bit Location + Width  bit1=-18  base1=MSB of Input  bit0=0  base0=LSB of Input  dbl_ovrd=off  block_type=slice
      settings: infoedit="Extracts a given range of bits from each input sample and presents it at the output.  The output type is ordinarily unsigned with binary point at zero, but can be Boolean when the slice is one bit wide.<P><P>Hardware notes: In hardware this block costs nothing."  block_version=10.1.2
  Slice3 : xbsIndex_r4/Slice  nbits=18  boolean_output=off  mode=Upper Bit Location + Width  bit1=-36  base1=MSB of Input  bit0=0  base0=LSB of Input  dbl_ovrd=off  block_type=slice
      settings: infoedit="Extracts a given range of bits from each input sample and presents it at the output.  The output type is ordinarily unsigned with binary point at zero, but can be Boolean when the slice is one bit wide.<P><P>Hardware notes: In hardware this block costs nothing."  block_version=10.1.2
  Slice4 : xbsIndex_r4/Slice  nbits=18  boolean_output=off  mode=Upper Bit Location + Width  bit1=-54  base1=MSB of Input  bit0=0  base0=LSB of Input  dbl_ovrd=off  block_type=slice
      settings: infoedit="Extracts a given range of bits from each input sample and presents it at the output.  The output type is ordinarily unsigned with binary point at zero, but can be Boolean when the slice is one bit wide.<P><P>Hardware notes: In hardware this block costs nothing."  block_version=10.1.2
  Out1 : Outport  OutDataType=sfix(16)  OutScaling=2^0
  Out2 : Outport  Port=2  OutDataType=sfix(16)  OutScaling=2^0
  Out3 : Outport  Port=3
  Out4 : Outport  Port=4
  wires:
  Reinterp4/1 -> Out4/1
  Slice4/1 -> Reinterp4/1
  Reinterp3/1 -> Out3/1
  Slice3/1 -> Reinterp3/1
  Reinterp2/1 -> Out2/1
  Slice2/1 -> Reinterp2/1
  Reinterp1/1 -> Out1/1
  Slice1/1 -> Reinterp1/1
  In/1 -> Slice4/1, Slice3/1, Slice2/1, Slice1/1

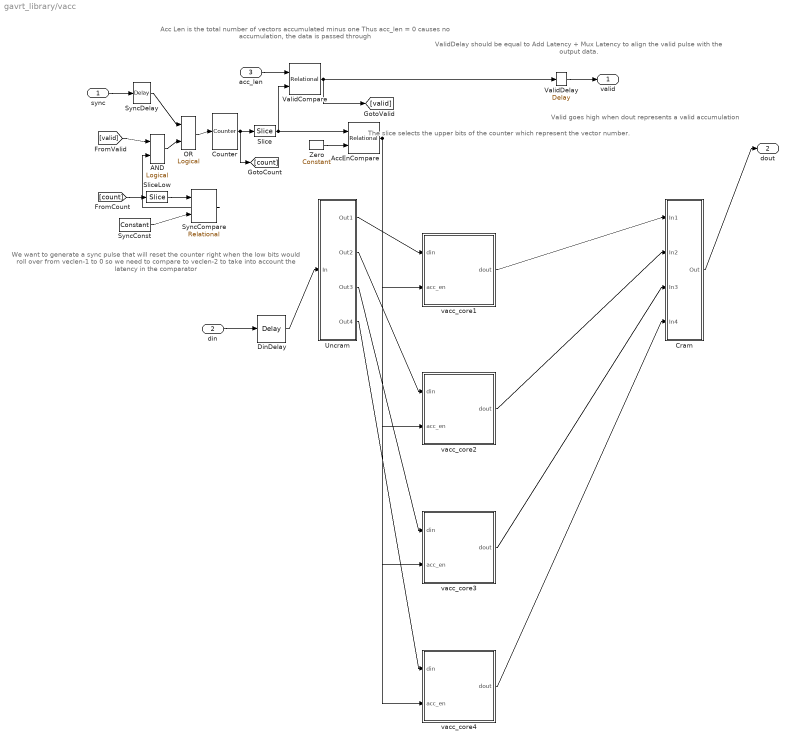
== system gavrt_library/vacc ==
  note: We want to generate a sync pulse that
      | will reset the counter right when the low bits
      | would roll over from veclen-1 to 0 so we need
      | to compare to veclen-2 to take into account
      | the latency in the comparator
  note: ValidDelay should be equal to
      | Add Latency + Mux Latency to align the valid pulse with the output data.
  note: Valid goes high when dout
      | represents a valid accumulation
  note: Acc Len is the total number of vectors accumulated minus one
      | Thus acc_len = 0 causes no accumulation, the data is passed through
  note: The slice selects the upper bits of the
      | counter which represent the vector number.
  sync : Inport  OutDataType=sfix(16)  OutScaling=2^0
  din : Inport  Port=2  OutDataType=sfix(16)  OutScaling=2^0
  acc_len : Inport  Port=3  OutDataType=sfix(16)  OutScaling=2^0
  AND : xbsIndex_r4/Logical  logical_function=AND  inputs=2  en=off  latency=0  precision=Full  arith_type=Unsigned  n_bits=8  bin_pt=2  align_bp=on  dbl_ovrd=off  block_type=logical
      settings: xl_area=[0, 0, 0, 0, 0, 0, 0]  block_version=10.1.2
  AccEnCompare : xbsIndex_r4/Relational  mode=a!=b  en=off  latency=1  dbl_ovrd=off  block_type=relational
      settings: xl_area=[0, 0, 0, 0, 0, 0, 0]  block_version=10.1.2
  Counter : xbsIndex_r4/Counter  cnt_type=Free Running  cnt_to=Inf  operation=Up  start_count=0  cnt_by_val=1  arith_type=Unsigned  n_bits=10  bin_pt=0  load_pin=off  rst=on  en=off  explicit_period=on  period=1  dbl_ovrd=off  use_behavioral_HDL=off  use_rpm=on  block_type=counter
      settings: xl_area=[0, 0, 0, 0, 0, 0, 0]  block_version=10.1.2
  Cram : Subsystem  AncestorBlock=gavrt_library/cram  mask(cram){num_slice=4}
      mask prompts: num_slice "Number of slices"
      mask help: Concatenates inputs together after forcing binary point to zero.
      mask init:
      | cram_init(gcb, ...
      |     'num_slice', num_slice);
  DinDelay : xbsIndex_r4/Delay  en=off  latency=2  dbl_ovrd=off  reg_retiming=off  block_type=delay
      settings: block_version=10.1.2
  OR : xbsIndex_r4/Logical  logical_function=OR  inputs=2  en=off  latency=0  precision=Full  arith_type=Unsigned  n_bits=8  bin_pt=2  align_bp=on  dbl_ovrd=off  block_type=logical
      settings: xl_area=[0, 0, 0, 0, 0, 0, 0]  block_version=10.1.2
  Slice : xbsIndex_r4/Slice  nbits=5  boolean_output=off  mode=Upper Bit Location + Width  bit1=0  base1=MSB of Input  bit0=0  base0=LSB of Input  dbl_ovrd=off  block_type=slice
      settings: infoedit="Extracts a given range of bits from each input sample and presents it at the output.  The output type is ordinarily unsigned with binary point at zero, but can be Boolean when the slice is one bit wide.<P><P>Hardware notes: In hardware this block costs nothing."  block_version=10.1.2
  SliceLow : xbsIndex_r4/Slice  nbits=5  boolean_output=off  mode=Lower Bit Location + Width  bit1=0  base1=MSB of Input  bit0=0  base0=LSB of Input  dbl_ovrd=off  block_type=slice
      settings: infoedit="Extracts a given range of bits from each input sample and presents it at the output.  The output type is ordinarily unsigned with binary point at zero, but can be Boolean when the slice is one bit wide.<P><P>Hardware notes: In hardware this block costs nothing."  block_version=10.1.2
  SyncCompare : xbsIndex_r4/Relational  mode=a=b  en=off  latency=1  dbl_ovrd=off  block_type=relational
      settings: xl_area=[0, 0, 0, 0, 0, 0, 0]  block_version=10.1.2
  SyncConst : xbsIndex_r4/Constant  arith_type=Unsigned  const=30  n_bits=5  bin_pt=0  explicit_period=on  period=1  equ=P=C  opselect=C  inp2=PCIN>>17  opr=+  inp1=P  carry=CIN  dbl_ovrd=off  block_type=constant
      settings: block_version=10.1.2
  SyncDelay : xbsIndex_r4/Delay  en=off  latency=0  dbl_ovrd=off  reg_retiming=off  block_type=delay
      settings: xl_area=[0, 0, 0, 0, 0, 0, 0]  block_version=10.1.2
  Uncram : Subsystem  AncestorBlock=gavrt_library/uncram  mask(uncram){num_slice=4, slice_width=18, bin_pt=17, arith_type=0}
      mask prompts: num_slice "Number of slices"; slice_width "Slice Width"; bin_pt "Output Binary Point"; arith_type "Output Arithmetic Type (0=Unsigned, 1=Signed, 2=Boolean)"
      mask help: Takes a concatenated input and slices it up into even pieces and reinterprets them as signed fixed point numbers with a given binary point.
      mask init:
      | uncram_init(gcb, ...
      |     'num_slice', num_slice, ...
      |     'slice_width', slice_width, ...
      |     'bin_pt', bin_pt, ...
      |     'arith_type', arith_type);
      settings: AttributesFormatString=UFix_18_17
  ValidCompare : xbsIndex_r4/Relational  mode=a=b  en=off  latency=1  dbl_ovrd=off  block_type=relational
      settings: xl_area=[0, 0, 0, 0, 0, 0, 0]  block_version=10.1.2
  ValidDelay : xbsIndex_r4/Delay  en=off  latency=3  dbl_ovrd=off  reg_retiming=off  block_type=delay
      settings: xl_area=[0, 0, 0, 0, 0, 0, 0]  block_version=10.1.2
  Zero : xbsIndex_r4/Constant  arith_type=Unsigned  const=0  n_bits=8  bin_pt=0  explicit_period=on  period=1  equ=P=C  opselect=C  inp2=PCIN>>17  opr=+  inp1=P  carry=CIN  dbl_ovrd=off  block_type=constant
      settings: block_version=10.1.2
  vacc_core1 : Subsystem  AncestorBlock=gavrt_library/vacc_core  mask(vacc_core){veclen=32, arith_type=0, out_bit_width=32, out_bin_pt=17, add_latency=2, bram_latency=2, mux_latency=1}
      mask prompts: veclen "Vector Length"; arith_type "Arithmetic Type (0=Unsigned, 1=Signed)"; out_bit_width "Output Bit Width"; out_bin_pt "Output Binary Point"; add_latency "Add Latency"; bram_latency "BRAM Latency"; mux_latency "Mux Latency"
      mask help:
      | Currently only Signed arithmetic supported
      | acc_en = 0 --> Load a vector (start a new accumulation)
      | acc_en = 1 --> Accumulate
      mask init: same as gavrt_library/vacc_core
  vacc_core2 : Subsystem  AncestorBlock=gavrt_library/vacc_core  mask(vacc_core){veclen=32, arith_type=0, out_bit_width=32, out_bin_pt=17, add_latency=2, bram_latency=2, mux_latency=1}
      mask prompts: veclen "Vector Length"; arith_type "Arithmetic Type (0=Unsigned, 1=Signed)"; out_bit_width "Output Bit Width"; out_bin_pt "Output Binary Point"; add_latency "Add Latency"; bram_latency "BRAM Latency"; mux_latency "Mux Latency"
      mask help:
      | Currently only Signed arithmetic supported
      | acc_en = 0 --> Load a vector (start a new accumulation)
      | acc_en = 1 --> Accumulate
      mask init: same as gavrt_library/vacc_core
  vacc_core3 : Subsystem  AncestorBlock=gavrt_library/vacc_core  mask(vacc_core){veclen=32, arith_type=0, out_bit_width=32, out_bin_pt=17, add_latency=2, bram_latency=2, mux_latency=1}
      mask prompts: veclen "Vector Length"; arith_type "Arithmetic Type (0=Unsigned, 1=Signed)"; out_bit_width "Output Bit Width"; out_bin_pt "Output Binary Point"; add_latency "Add Latency"; bram_latency "BRAM Latency"; mux_latency "Mux Latency"
      mask help:
      | Currently only Signed arithmetic supported
      | acc_en = 0 --> Load a vector (start a new accumulation)
      | acc_en = 1 --> Accumulate
      mask init: same as gavrt_library/vacc_core
  vacc_core4 : Subsystem  AncestorBlock=gavrt_library/vacc_core  mask(vacc_core){veclen=32, arith_type=0, out_bit_width=32, out_bin_pt=17, add_latency=2, bram_latency=2, mux_latency=1}
      mask prompts: veclen "Vector Length"; arith_type "Arithmetic Type (0=Unsigned, 1=Signed)"; out_bit_width "Output Bit Width"; out_bin_pt "Output Binary Point"; add_latency "Add Latency"; bram_latency "BRAM Latency"; mux_latency "Mux Latency"
      mask help:
      | Currently only Signed arithmetic supported
      | acc_en = 0 --> Load a vector (start a new accumulation)
      | acc_en = 1 --> Accumulate
      mask init: same as gavrt_library/vacc_core
  valid : Outport  OutDataType=sfix(16)  OutScaling=2^0
  dout : Outport  Port=2  OutDataType=sfix(16)  OutScaling=2^0
  wires:
  vacc_core4/1(dout) -> Cram/4(In4)
  Uncram/4(Out4) -> vacc_core4/1(din)
  vacc_core3/1(dout) -> Cram/3(In3)
  Uncram/3(Out3) -> vacc_core3/1(din)
  vacc_core2/1(dout) -> Cram/2(In2)
  Uncram/2(Out2) -> vacc_core2/1(din)
  vacc_core1/1(dout) -> Cram/1(In1)
  AccEnCompare/1 -> vacc_core4/2(acc_en), vacc_core3/2(acc_en), vacc_core2/2(acc_en), vacc_core1/2(acc_en)
  Uncram/1(Out1) -> vacc_core1/1(din)
  Cram/1(Out) -> dout/1
  DinDelay/1 -> Uncram/1(In)
  din/1 -> DinDelay/1
  ValidDelay/1 -> valid/1
  Zero/1 -> AccEnCompare/2
  Slice/1 -> AccEnCompare/1, ValidCompare/2
  acc_len/1 -> ValidCompare/1
  ValidCompare/1 -> ValidDelay/1, [valid]
  SyncCompare/1 -> AND/2
  SyncConst/1 -> SyncCompare/2
  SliceLow/1 -> SyncCompare/1
  [count] -> SliceLow/1
  Counter/1 -> Slice/1, [count]
  OR/1 -> Counter/1
  AND/1 -> OR/2
  [valid] -> AND/1
  SyncDelay/1 -> OR/1
  sync/1 -> SyncDelay/1

== system gavrt_library/vacc_core ==
  note: This BRAM and counter is exactly what is inside the green
      | Delay BRAM block. The functionality was extracted to avoid
      | library issues.
  din : Inport  OutDataType=sfix(16)  OutScaling=2^0
  acc_en : Inport  Port=2  OutDataType=sfix(16)  OutScaling=2^0
  Adder : xbsIndex_r4/AddSub  mode=Addition  use_carryin=off  use_carryout=off  en=off  latency=2  precision=User Defined  arith_type="Signed  (2's comp)"  n_bits=32  bin_pt=7  quantization=Truncate  overflow=Wrap  dbl_ovrd=off  use_behavioral_HDL=on  pipelined=on  use_rpm=on  block_type=addsub
      settings: xl_area=[0, 0, 0, 0, 0, 0, 0]  block_version=10.1.2
  BRAM : xbsIndex_r4/Single Port RAM  depth=32  initVector=0  distributed_mem=Block RAM  write_mode=Read Before Write  rst=off  init_reg=0  en=off  latency=2  dbl_ovrd=off  optimize=Area  use_rpm=off  block_type=spram
      settings: xl_area=[0, 0, 0, 0, 0, 0, 0]  block_version=10.1.2
  Constant : xbsIndex_r4/Constant  arith_type=Unsigned  const=0  n_bits=1  bin_pt=0  explicit_period=off  period=1  equ=P=C  opselect=C  inp2=PCIN>>17  opr=+  inp1=P  carry=CIN  dbl_ovrd=off  block_type=constant
      settings: block_version=10.1.2
  Constant2 : xbsIndex_r4/Constant  arith_type=Boolean  const=1  n_bits=1  bin_pt=0  explicit_period=on  period=1  equ=P=C  opselect=C  inp2=PCIN>>17  opr=+  inp1=P  carry=CIN  dbl_ovrd=off  block_type=constant
      settings: block_version=10.1.2
  Counter : xbsIndex_r4/Counter  cnt_type=Count Limited  cnt_to=27  operation=Up  start_count=0  cnt_by_val=1  arith_type=Unsigned  n_bits=5  bin_pt=0  load_pin=off  rst=off  en=off  explicit_period=off  period=1  dbl_ovrd=off  use_behavioral_HDL=off  use_rpm=off  block_type=counter
      settings: xl_area=[0, 0, 0, 0, 0, 0, 0]  block_version=10.1.2
  Mux : xbsIndex_r4/Mux  inputs=2  en=off  latency=0  precision=Full  arith_type="Signed  (2's comp)"  n_bits=8  bin_pt=2  quantization=Truncate  overflow=Wrap  dbl_ovrd=off  block_type=mux
      settings: xl_area=[0, 0, 0, 0, 0, 0, 0]  block_version=10.1.2
  warn period Adder0 : xbsReplacements_r4/Warning  SystemSampleTime=-1  period=1
  dout : Outport  OutDataType=sfix(16)  OutScaling=2^0
  wires:
  Constant2/1 -> BRAM/3
  Counter/1 -> BRAM/1
  Adder/1 -> BRAM/2, dout/1
  Mux/1 -> Adder/2
  din/1 -> Adder/1
  BRAM/1 -> Mux/3
  Constant/1 -> Mux/2
  acc_en/1 -> Mux/1

== system gavrt_library/DataRateChanger/Uncram ==
  In : Inport  OutDataType=sfix(16)  OutScaling=2^0
  Reinterp1 : xbsIndex_r4/Reinterpret  force_arith_type=on  arith_type=Unsigned  force_bin_pt=on  bin_pt=0  block_type=reinterpret
      settings: infoedit="Changes signal type without altering the binary representation.   You can changed the signal between signed and unsigned, and relocate the binary point.<P><P>Hardware notes: In hardware this block costs nothing.<P><P>Example:  Suppose the input is 6 bits wide, signed, with 2 fractional bits, and the output is forced to unsigned with 0 fractional bits.  Then an input of -2.0 (1110.00 in binary 2's complement) becomes an output of 56 (111000 in binary)."  block_version=10.1.2
  Reinterp2 : xbsIndex_r4/Reinterpret  force_arith_type=on  arith_type=Unsigned  force_bin_pt=on  bin_pt=0  block_type=reinterpret
      settings: infoedit="Changes signal type without altering the binary representation.   You can changed the signal between signed and unsigned, and relocate the binary point.<P><P>Hardware notes: In hardware this block costs nothing.<P><P>Example:  Suppose the input is 6 bits wide, signed, with 2 fractional bits, and the output is forced to unsigned with 0 fractional bits.  Then an input of -2.0 (1110.00 in binary 2's complement) becomes an output of 56 (111000 in binary)."  block_version=10.1.2
  Slice1 : xbsIndex_r4/Slice  nbits=8  boolean_output=off  mode=Upper Bit Location + Width  bit1=0  base1=MSB of Input  bit0=0  base0=LSB of Input  dbl_ovrd=off  block_type=slice
      settings: infoedit="Extracts a given range of bits from each input sample and presents it at the output.  The output type is ordinarily unsigned with binary point at zero, but can be Boolean when the slice is one bit wide.<P><P>Hardware notes: In hardware this block costs nothing."  block_version=10.1.2
  Slice2 : xbsIndex_r4/Slice  nbits=8  boolean_output=off  mode=Upper Bit Location + Width  bit1=-8  base1=MSB of Input  bit0=0  base0=LSB of Input  dbl_ovrd=off  block_type=slice
      settings: infoedit="Extracts a given range of bits from each input sample and presents it at the output.  The output type is ordinarily unsigned with binary point at zero, but can be Boolean when the slice is one bit wide.<P><P>Hardware notes: In hardware this block costs nothing."  block_version=10.1.2
  Out1 : Outport  OutDataType=sfix(16)  OutScaling=2^0
  Out2 : Outport  Port=2
  wires:
  Reinterp2/1 -> Out2/1
  Slice2/1 -> Reinterp2/1
  Reinterp1/1 -> Out1/1
  Slice1/1 -> Reinterp1/1
  In/1 -> Slice2/1, Slice1/1

== system gavrt_library/DataRateChanger/freeze_cntr ==
  en : Inport  OutDataType=sfix(16)  OutScaling=2^0
  rst : Inport  Port=2  OutDataType=sfix(16)  OutScaling=2^0
  Counter3 : xbsIndex_r4/Counter  cnt_type=Free Running  cnt_to=1023  operation=Up  start_count=0  cnt_by_val=1  arith_type=Unsigned  n_bits=CounterBits + 1  bin_pt=0  load_pin=off  rst=on  en=on  explicit_period=on  period=1  dbl_ovrd=off  use_behavioral_HDL=off  use_rpm=on  block_type=counter
      settings: xl_area=[0, 0, 0, 0, 0, 0, 0]  block_version=10.1.2
  Inverter : xbsIndex_r4/Inverter  en=off  latency=0  dbl_ovrd=off  block_type=inv
      settings: xl_area=[0, 0, 0, 0, 0, 0, 0]  block_version=10.1.2
  Inverter1 : xbsIndex_r4/Inverter  en=off  latency=0  dbl_ovrd=off  block_type=inv
      settings: xl_area=[0, 0, 0, 0, 0, 0, 0]  block_version=10.1.2
  Logical1 : xbsIndex_r4/Logical  logical_function=AND  inputs=2  en=off  latency=0  precision=Full  arith_type=Unsigned  n_bits=8  bin_pt=2  align_bp=on  dbl_ovrd=off  block_type=logical
      settings: xl_area=[0, 0, 0, 0, 0, 0, 0]  block_version=10.1.2
  Logical5 : xbsIndex_r4/Logical  logical_function=AND  inputs=2  en=off  latency=0  precision=Full  arith_type=Unsigned  n_bits=8  bin_pt=2  align_bp=on  dbl_ovrd=off  block_type=logical
      settings: xl_area=[0, 0, 0, 0, 0, 0, 0]  block_version=10.1.2
  enable : xbsIndex_r4/Slice  nbits=CounterBits  boolean_output=off  mode=Lower Bit Location + Width  bit1=0  base1=LSB of Input  bit0=0  base0=LSB of Input  dbl_ovrd=off  block_type=slice
      settings: infoedit="Extracts a given range of bits from each input sample and presents it at the output.  The output type is ordinarily unsigned with binary point at zero, but can be Boolean when the slice is one bit wide.<P><P>Hardware notes: In hardware this block costs nothing."  block_version=10.1.2
  enable1 : xbsIndex_r4/Slice  nbits=1  boolean_output=on  mode=Upper Bit Location + Width  bit1=0  base1=MSB of Input  bit0=0  base0=LSB of Input  dbl_ovrd=off  block_type=slice
      settings: infoedit="Extracts a given range of bits from each input sample and presents it at the output.  The output type is ordinarily unsigned with binary point at zero, but can be Boolean when the slice is one bit wide.<P><P>Hardware notes: In hardware this block costs nothing."  block_version=10.1.2
  addr : Outport  OutDataType=sfix(16)  OutScaling=2^0
  we : Outport  Port=2  OutDataType=sfix(16)  OutScaling=2^0
  done : Outport  Port=3  OutDataType=sfix(16)  OutScaling=2^0
  wires:
  Inverter1/1 -> Logical5/2
  enable/1 -> addr/1
  rst/1 -> Counter3/1, Inverter/1
  Logical5/1 -> Counter3/2, Logical1/2
  en/1 -> Logical5/1
  enable1/1 -> done/1, Inverter1/1
  Counter3/1 -> enable/1, enable1/1
  Inverter/1 -> Logical1/1
  Logical1/1 -> we/1
